simulink model "model_5_4"  (R2020a)
settings: Solver=VariableStepAuto  StartTime=0.0  StopTime=10.0  RelTol=1e-3
settings Model: Creator=Shadman  LastModifiedBy=Shadman

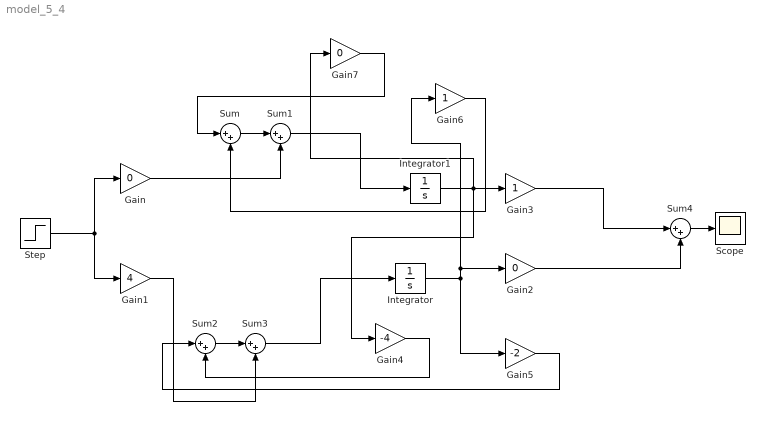
== system model_5_4 ==
  Gain : Gain  Gain=0
  Gain1 : Gain  Gain=4
  Gain2 : Gain  Gain=0
  Gain3 : Gain
  Gain4 : Gain  Gain=-4
  Gain5 : Gain  Gain=-2
  Gain6 : Gain
  Gain7 : Gain  Gain=0
  Integrator : Integrator
  Integrator1 : Integrator
  Scope : Scope
  Step : Step  Time=0  SampleTime=0
  Sum{,1..4} (5 alike) : Sum  Inputs=|++
  wires:
  Step/1 -> Gain1/1, Gain/1
  Sum/1 -> Sum1/1
  Sum2/1 -> Sum3/1
  Gain4/1 -> Sum2/2
  Gain1/1 -> Sum3/2
  Gain5/1 -> Sum2/1
  Sum4/1 -> Scope/1
  Gain3/1 -> Sum4/1
  Gain2/1 -> Sum4/2
  Integrator/1 -> Gain6/1, Gain2/1, Gain5/1
  Gain6/1 -> Sum/2
  Gain7/1 -> Sum/1
  Integrator1/1 -> Gain4/1, Gain7/1, Gain3/1
  Sum1/1 -> Integrator1/1
  Gain/1 -> Sum1/2
  Sum3/1 -> Integrator/1
